simulink library "avionics_S2_lib"  (Simulink 6.6)
undefined symbols (not defined in the file or in its folder): AirData, EngineID, MAG3, Pots, Timestep, Vanes
libraries: aeroutilslib x3, Telemetry_Lib x3, Calibration_Lib x2, simulink x1
settings Model: Creator=amurch  LastModifiedBy=amurch

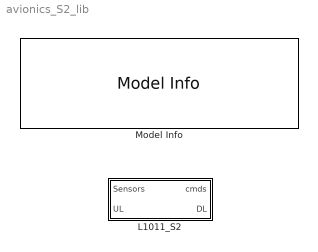
== system avionics_S2_lib ==
  L1011_S2 : Subsystem
  Model Info : simulink/Model-Wide Utilities/Model Info  SystemSampleTime=-1  InitialBlockCM=None  BlockCM=None  Frame=on  DisplayStringWithTags=|  HorizontalTextAlignment=Center  LeftAlignmentValue=0.5  SourceBlockDiagram=avionics_S2_lib  TagMaxNumber=20
      | L1011 S2 Avionics Library
      | %<ModelVersion>
      | Las modified by %<LastModifiedBy> on %<LastModificationDate>

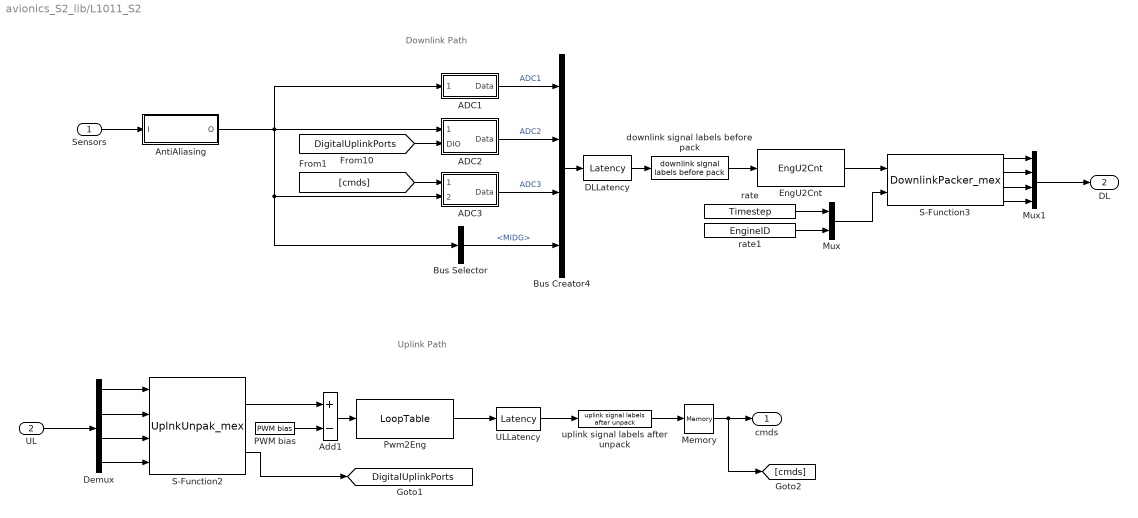
== system avionics_S2_lib/L1011_S2 ==
  note: Uplink Path
  note: Downlink Path
  Sensors : Inport
  UL : Inport  Port=2
  ADC1 : Subsystem
  ADC2 : Subsystem
  ADC3 : Subsystem
  Add1 : Sum  Inputs=+-  OutScaling=2^-10
  AntiAliasing : Subsystem
  Bus Creator4 : BusCreator
  Bus Selector : BusSelector  OutputSignals=MIDG
  DLLatency : aeroutilslib/Latency  SystemSampleTime=-1  Latency=.01  timestep=Timestep
  Demux : Demux
  EngU2Cnt : Calibration_Lib/EngU2Cnt  SystemSampleTime=-1
  Memory : Memory
  Mux : Mux  Inputs=2
  Mux1 : Mux
  PWM bias : Telemetry_Lib/PWM bias  SystemSampleTime=-1
  Pwm2Eng : Calibration_Lib/LoopTable  SystemSampleTime=-1  XTable=UpCals_Pwm  YTable=UpCals_Eng
  S-Function2 : S-Function  FunctionName=UplnkUnpak_mex
  S-Function3 : S-Function  FunctionName=DownlinkPacker_mex
  ULLatency : aeroutilslib/Latency  SystemSampleTime=-1  Latency=.01  timestep=Timestep
  downlink signal labels before pack : Telemetry_Lib/downlink signal labels before pack  SystemSampleTime=-1
  rate : Constant  Value=Timestep
  rate1 : Constant  Value=EngineID
  uplink signal labels after unpack : Telemetry_Lib/uplink signal labels after unpack  SystemSampleTime=-1
  cmds : Outport
  DL : Outport  Port=2
  tag scope: DigitalUplinkPorts=global
  wires:
  Sensors/1 -> AntiAliasing/1(I)
  EngU2Cnt/1 -> S-Function3/1
  rate/1 -> Mux/1
  rate1/1 -> Mux/2
  Mux/1 -> S-Function3/2
  S-Function3/1 -> Mux1/1
  S-Function3/2 -> Mux1/2
  S-Function3/3 -> Mux1/3
  S-Function3/4 -> Mux1/4
  Mux1/1 -> DL/1
  S-Function2/2 -> [DigitalUplinkPorts]
  Pwm2Eng/1 -> ULLatency/1
  uplink signal labels after unpack/1 -> Memory/1
  Demux/1 -> S-Function2/1
  Demux/2 -> S-Function2/2
  Demux/3 -> S-Function2/3
  Demux/4 -> S-Function2/4
  UL/1 -> Demux/1
  ADC1/1(Data) -> Bus Creator4/1  "ADC1"
  ADC2/1(Data) -> Bus Creator4/2  "ADC2"
  ADC3/1(Data) -> Bus Creator4/3  "ADC3"
  AntiAliasing/1(O) -> ADC1/1(ADC1), ADC2/1(ADC2), ADC3/2(ADC3), Bus Selector/1
  Bus Selector/1 -> Bus Creator4/4  "<MIDG>"
  Bus Creator4/1 -> DLLatency/1
  Memory/1 -> cmds/1, [cmds]
  ULLatency/1 -> uplink signal labels after unpack/1
  downlink signal labels before pack/1 -> EngU2Cnt/1
  DLLatency/1 -> downlink signal labels before pack/1
  [DigitalUplinkPorts] -> ADC2/2(DIO)
  [cmds] -> ADC3/1(cmds)
  PWM bias/1 -> Add1/2
  Add1/1 -> Pwm2Eng/1
  S-Function2/1 -> Add1/1

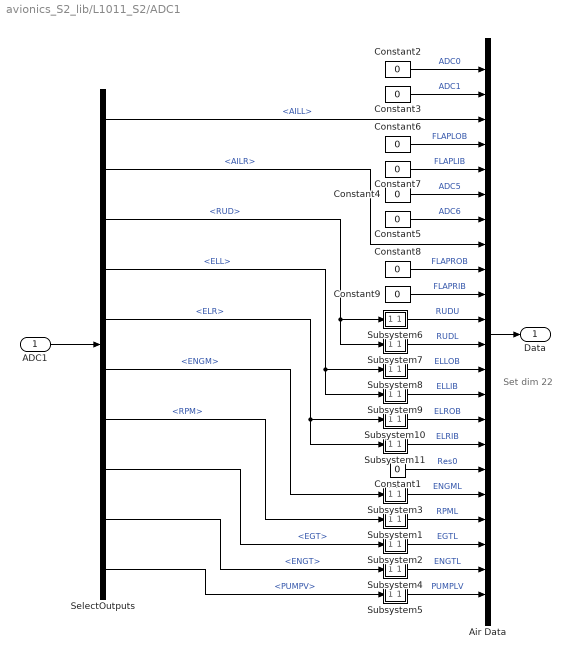
== system avionics_S2_lib/L1011_S2/ADC1 ==
  note: Set dim 22
  ADC1 : Inport
  Air Data : BusCreator  Inputs=22
  Constant{1..9} (9 alike) : Constant  Value=0
  SelectOutputs : BusSelector  OutputSignals=Pots.AILL,Pots.AILR,Pots.RUD,Pots.ELL,Pots.ELR,ECU.ENGM,ECU.RPM,ECU.EGT,ECU.ENGT,ECU.PUMPV
  Subsystem1 : Subsystem
  Subsystem10 : Subsystem
  Subsystem11 : Subsystem
  Subsystem2 : Subsystem
  Subsystem3 : Subsystem
  Subsystem4 : Subsystem
  Subsystem5 : Subsystem
  Subsystem6 : Subsystem
  Subsystem7 : Subsystem
  Subsystem8 : Subsystem
  Subsystem9 : Subsystem
  Data : Outport  PortDimensions=22
  wires:
  Constant1/1 -> Air Data/17  "Res0"
  Air Data/1 -> Data/1
  ADC1/1 -> SelectOutputs/1
  Constant2/1 -> Air Data/1  "ADC0"
  Constant3/1 -> Air Data/2  "ADC1"
  Constant4/1 -> Air Data/6  "ADC5"
  Constant5/1 -> Air Data/7  "ADC6"
  SelectOutputs/1 -> Air Data/3  "<AILL>"
  SelectOutputs/2 -> Air Data/8  "<AILR>"
  SelectOutputs/6 -> Subsystem3/1(I)  "<ENGM>"
  SelectOutputs/7 -> Subsystem1/1(I)  "<RPM>"
  SelectOutputs/8 -> Subsystem2/1(I)  "<EGT>"
  SelectOutputs/9 -> Subsystem4/1(I)  "<ENGT>"
  SelectOutputs/10 -> Subsystem5/1(I)  "<PUMPV>"
  Subsystem3/1(O) -> Air Data/18  "ENGML"
  Subsystem1/1(O) -> Air Data/19  "RPML"
  Subsystem2/1(O) -> Air Data/20  "EGTL"
  Subsystem4/1(O) -> Air Data/21  "ENGTL"
  Subsystem5/1(O) -> Air Data/22  "PUMPLV"
  Constant6/1 -> Air Data/4  "FLAPLOB"
  Constant7/1 -> Air Data/5  "FLAPLIB"
  Constant8/1 -> Air Data/9  "FLAPROB"
  Constant9/1 -> Air Data/10  "FLAPRIB"
  Subsystem6/1(O) -> Air Data/11  "RUDU"
  Subsystem7/1(O) -> Air Data/12  "RUDL"
  Subsystem8/1(O) -> Air Data/13  "ELLOB"
  Subsystem9/1(O) -> Air Data/14  "ELLIB"
  Subsystem10/1(O) -> Air Data/15  "ELROB"
  Subsystem11/1(O) -> Air Data/16  "ELRIB"
  SelectOutputs/3 -> Subsystem6/1(I), Subsystem7/1(I)  "<RUD>"
  SelectOutputs/4 -> Subsystem8/1(I), Subsystem9/1(I)  "<ELL>"
  SelectOutputs/5 -> Subsystem10/1(I), Subsystem11/1(I)  "<ELR>"

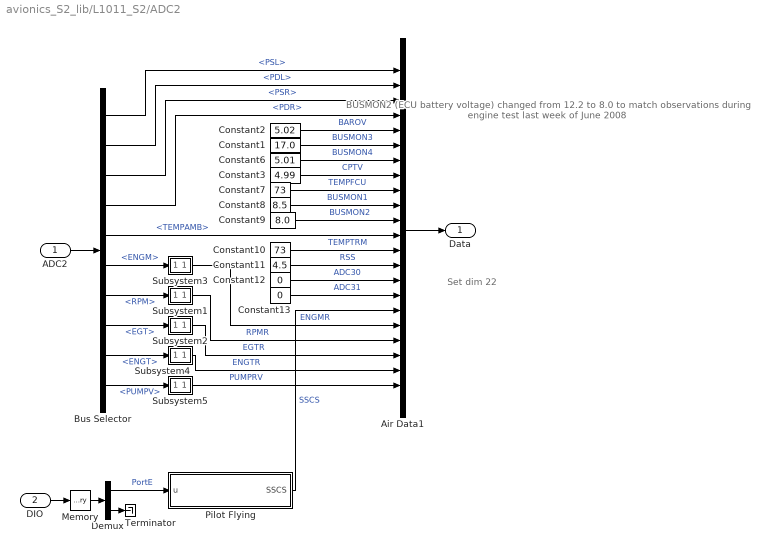
== system avionics_S2_lib/L1011_S2/ADC2 ==
  note: BUSMON2 (ECU battery voltage)
      | changed from 12.2 to 8.0 to
      | match observations during engine test
      | last week of June 2008
  note: Set dim 22
  ADC2 : Inport
  DIO : Inport  Port=2
  Air Data1 : BusCreator  Inputs=22
  Bus Selector : BusSelector  OutputSignals=AirData.PSL,AirData.PDL,AirData.PSR,AirData.PDR,AirData.TEMPAMB,ECU.ENGM,ECU.RPM,ECU.EGT,ECU.ENGT,ECU.PUMPV
  Constant1 : Constant  Value=17.0
  Constant10 : Constant  Value=73
  Constant11 : Constant  Value=4.5
  Constant12 : Constant  Value=0
  Constant13 : Constant  Value=0
  Constant2 : Constant  Value=5.02
  Constant3 : Constant  Value=4.99
  Constant6 : Constant  Value=5.01
  Constant7 : Constant  Value=73
  Constant8 : Constant  Value=8.5
  Constant9 : Constant  Value=8.0
  Demux : Demux  Outputs=2
  Memory : Memory
  Pilot Flying : Stateflow chart
  Subsystem1 : Subsystem
  Subsystem2 : Subsystem
  Subsystem3 : Subsystem
  Subsystem4 : Subsystem
  Subsystem5 : Subsystem
  Terminator : Terminator
  Data : Outport  PortDimensions=22
  wires:
  Air Data1/1 -> Data/1
  ADC2/1 -> Bus Selector/1
  Bus Selector/1 -> Air Data1/1  "<PSL>"
  Bus Selector/2 -> Air Data1/2  "<PDL>"
  Bus Selector/3 -> Air Data1/3  "<PSR>"
  Bus Selector/4 -> Air Data1/4  "<PDR>"
  Bus Selector/5 -> Air Data1/12  "<TEMPAMB>"
  Bus Selector/6 -> Subsystem3/1(I)  "<ENGM>"
  Bus Selector/7 -> Subsystem1/1(I)  "<RPM>"
  Bus Selector/8 -> Subsystem2/1(I)  "<EGT>"
  Bus Selector/10 -> Subsystem5/1(I)  "<PUMPV>"
  Constant2/1 -> Air Data1/5  "BAROV"
  Constant1/1 -> Air Data1/6  "BUSMON3"
  Constant6/1 -> Air Data1/7  "BUSMON4"
  Constant3/1 -> Air Data1/8  "CPTV"
  Constant7/1 -> Air Data1/9  "TEMPFCU"
  Constant8/1 -> Air Data1/10  "BUSMON1"
  Constant9/1 -> Air Data1/11  "BUSMON2"
  Constant10/1 -> Air Data1/13  "TEMPTRM"
  Constant11/1 -> Air Data1/14  "RSS"
  Constant12/1 -> Air Data1/15  "ADC30"
  Constant13/1 -> Air Data1/16  "ADC31"
  Pilot Flying/1(SSCS) -> Air Data1/17  "SSCS"
  DIO/1 -> Memory/1
  Demux/2 -> Terminator/1
  Demux/1 -> Pilot Flying/1(u)  "PortE"
  Memory/1 -> Demux/1
  Bus Selector/9 -> Subsystem4/1(I)  "<ENGT>"
  Subsystem3/1(O) -> Air Data1/18  "ENGMR"
  Subsystem1/1(O) -> Air Data1/19  "RPMR"
  Subsystem2/1(O) -> Air Data1/20  "EGTR"
  Subsystem4/1(O) -> Air Data1/21  "ENGTR"
  Subsystem5/1(O) -> Air Data1/22  "PUMPRV"

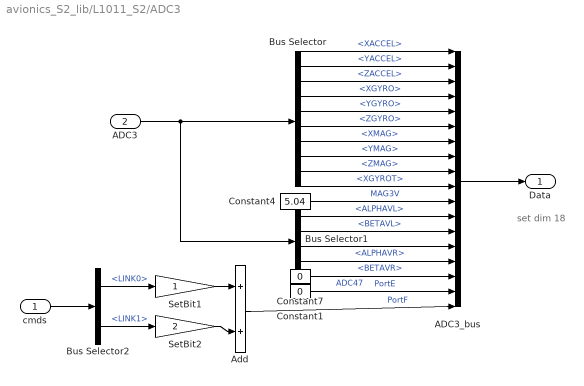
== system avionics_S2_lib/L1011_S2/ADC3 ==
  note: set dim 18
  cmds : Inport
  ADC3 : Inport  Port=2
  ADC3_bus : BusCreator  Inputs=18
  Add : Sum  OutScaling=2^-10
  Bus Selector : BusSelector  OutputSignals=MAG3.XACCEL,MAG3.YACCEL,MAG3.ZACCEL,MAG3.XGYRO,MAG3.YGYRO,MAG3.ZGYRO,MAG3.XMAG,MAG3.YMAG,MAG3.ZMAG,MAG3.XGYROT
  Bus Selector1 : BusSelector  OutputSignals=Vanes.ALPHAVL,Vanes.BETAVL,Vanes.ALPHAVR,Vanes.BETAVR
  Bus Selector2 : BusSelector  OutputSignals=LINK0,LINK1
  Constant1 : Constant  Value=0
  Constant4 : Constant  Value=5.04
  Constant7 : Constant  Value=0
  SetBit1 : Gain
  SetBit2 : Gain  Gain=2
  Data : Outport  PortDimensions=18
  wires:
  Add/1 -> ADC3_bus/18  "PortF"
  cmds/1 -> Bus Selector2/1
  Constant1/1 -> ADC3_bus/17  "PortE"
  ADC3_bus/1 -> Data/1
  ADC3/1 -> Bus Selector/1, Bus Selector1/1
  Constant4/1 -> ADC3_bus/11  "MAG3V"
  Bus Selector1/1 -> ADC3_bus/12  "<ALPHAVL>"
  Bus Selector1/2 -> ADC3_bus/13  "<BETAVL>"
  Bus Selector1/3 -> ADC3_bus/14  "<ALPHAVR>"
  Bus Selector1/4 -> ADC3_bus/15  "<BETAVR>"
  Constant7/1 -> ADC3_bus/16  "ADC47"
  Bus Selector/10 -> ADC3_bus/10  "<XGYROT>"
  Bus Selector/1 -> ADC3_bus/1  "<XACCEL>"
  Bus Selector/2 -> ADC3_bus/2  "<YACCEL>"
  Bus Selector/3 -> ADC3_bus/3  "<ZACCEL>"
  Bus Selector/4 -> ADC3_bus/4  "<XGYRO>"
  Bus Selector/5 -> ADC3_bus/5  "<YGYRO>"
  Bus Selector/6 -> ADC3_bus/6  "<ZGYRO>"
  Bus Selector/7 -> ADC3_bus/7  "<XMAG>"
  Bus Selector/8 -> ADC3_bus/8  "<YMAG>"
  Bus Selector/9 -> ADC3_bus/9  "<ZMAG>"
  Bus Selector2/1 -> SetBit1/1  "<LINK0>"
  Bus Selector2/2 -> SetBit2/1  "<LINK1>"
  SetBit1/1 -> Add/1
  SetBit2/1 -> Add/2

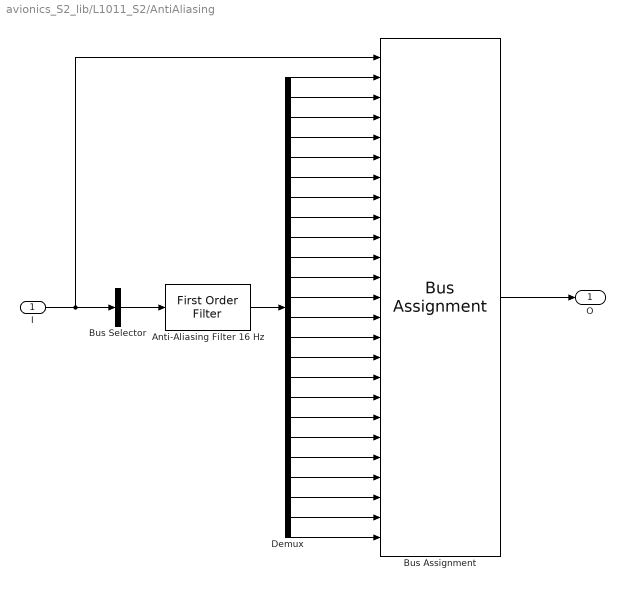
== system avionics_S2_lib/L1011_S2/AntiAliasing ==
  I : Inport
  Anti-Aliasing Filter 16 Hz : aeroutilslib/First Order Filter  SystemSampleTime=-1  tau=1/(32*pi)  timestep=Timestep
  Bus Assignment : BusAssignment  AssignedSignals=Vanes.ALPHAVL,Vanes.BETAVL,Vanes.ALPHAVR,Vanes.BETAVR,AirData.PDL,AirData.PSL,AirData.PDR,AirData.PSR,AirData.TEMPAMB,MAG3.XMAG,MAG3.YMAG,MAG3.ZMAG,MAG3.XGYRO,MAG3.YGYRO,MAG3.ZGYRO,MAG3.XACCEL,MAG3.YACCEL,MAG3.ZACCEL,MAG3.XGYROT,Pots.ELL,Pots.ELR,Pots.AILL,Pots.AILR,Pots.RUD
  Bus Selector : BusSelector  OutputSignals=Vanes,AirData,MAG3,Pots  OutputAsBus=on
  Demux : Demux  Outputs=24
  O : Outport
  wires:
  I/1 -> Bus Selector/1, Bus Assignment/1
  Bus Selector/1 -> Anti-Aliasing Filter 16 Hz/1
  Anti-Aliasing Filter 16 Hz/1 -> Demux/1
  Demux/1 -> Bus Assignment/2
  Demux/2 -> Bus Assignment/3
  Demux/3 -> Bus Assignment/4
  Demux/4 -> Bus Assignment/5
  Demux/5 -> Bus Assignment/6
  Demux/6 -> Bus Assignment/7
  Demux/7 -> Bus Assignment/8
  Demux/8 -> Bus Assignment/9
  Demux/9 -> Bus Assignment/10
  Demux/10 -> Bus Assignment/11
  Demux/11 -> Bus Assignment/12
  Demux/12 -> Bus Assignment/13
  Demux/13 -> Bus Assignment/14
  Demux/14 -> Bus Assignment/15
  Demux/15 -> Bus Assignment/16
  Demux/16 -> Bus Assignment/17
  Demux/17 -> Bus Assignment/18
  Demux/18 -> Bus Assignment/19
  Demux/19 -> Bus Assignment/20
  Bus Assignment/1 -> O/1
  Demux/20 -> Bus Assignment/21
  Demux/21 -> Bus Assignment/22
  Demux/22 -> Bus Assignment/23
  Demux/23 -> Bus Assignment/24
  Demux/24 -> Bus Assignment/25

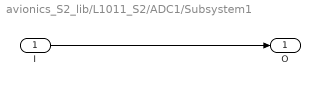
== system avionics_S2_lib/L1011_S2/ADC1/Subsystem1 ==
  I : Inport
  O : Outport
  wires:
  I/1 -> O/1

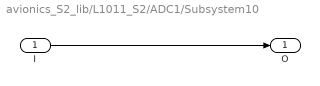
== system avionics_S2_lib/L1011_S2/ADC1/Subsystem10 ==
  I : Inport
  O : Outport
  wires:
  I/1 -> O/1

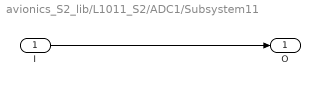
== system avionics_S2_lib/L1011_S2/ADC1/Subsystem11 ==
  I : Inport
  O : Outport
  wires:
  I/1 -> O/1

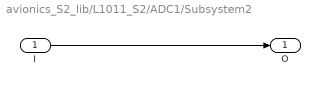
== system avionics_S2_lib/L1011_S2/ADC1/Subsystem2 ==
  I : Inport
  O : Outport
  wires:
  I/1 -> O/1

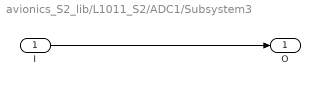
== system avionics_S2_lib/L1011_S2/ADC1/Subsystem3 ==
  I : Inport
  O : Outport
  wires:
  I/1 -> O/1

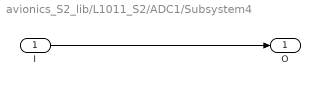
== system avionics_S2_lib/L1011_S2/ADC1/Subsystem4 ==
  I : Inport
  O : Outport
  wires:
  I/1 -> O/1

== system avionics_S2_lib/L1011_S2/ADC1/Subsystem5 ==
  I : Inport
  O : Outport
  wires:
  I/1 -> O/1

== system avionics_S2_lib/L1011_S2/ADC1/Subsystem6 ==
  I : Inport
  O : Outport
  wires:
  I/1 -> O/1

== system avionics_S2_lib/L1011_S2/ADC1/Subsystem7 ==
  I : Inport
  O : Outport
  wires:
  I/1 -> O/1

== system avionics_S2_lib/L1011_S2/ADC1/Subsystem8 ==
  I : Inport
  O : Outport
  wires:
  I/1 -> O/1

== system avionics_S2_lib/L1011_S2/ADC1/Subsystem9 ==
  I : Inport
  O : Outport
  wires:
  I/1 -> O/1

== system avionics_S2_lib/L1011_S2/ADC2/Subsystem1 ==
  I : Inport
  O : Outport
  wires:
  I/1 -> O/1

== system avionics_S2_lib/L1011_S2/ADC2/Subsystem2 ==
  I : Inport
  O : Outport
  wires:
  I/1 -> O/1

== system avionics_S2_lib/L1011_S2/ADC2/Subsystem3 ==
  I : Inport
  O : Outport
  wires:
  I/1 -> O/1

== system avionics_S2_lib/L1011_S2/ADC2/Subsystem4 ==
  I : Inport
  O : Outport
  wires:
  I/1 -> O/1

== system avionics_S2_lib/L1011_S2/ADC2/Subsystem5 ==
  I : Inport
  O : Outport
  wires:
  I/1 -> O/1

== matlab function L1011_S2/ADC2/Pilot Flying ==
  data: u input inherited; SSCS output inherited
function SSCS = setSSCS(u)
% This block supports an embeddable subset of the MATLAB language.
% See the help menu for details. 

SSCS = double(0);
RPf = uint8(0);
RPf = bitget(u,8);
if RPf==1
    SSCS = 6.0;  %research pilot flying (SSCS)
else
    SSCS = 4.0;  %safety pilot flying  (SSCS)
end
